simulink model "DVB_S2X_64APSK_Receiver_Sim"  (R2025b)
settings: Solver=VariableStepAuto  StartTime=0.0  StopTime=10.0  RelTol=1e-3
libraries: simulink x1
settings Model: Creator=vaggelis  LastModifiedBy=vaggelis

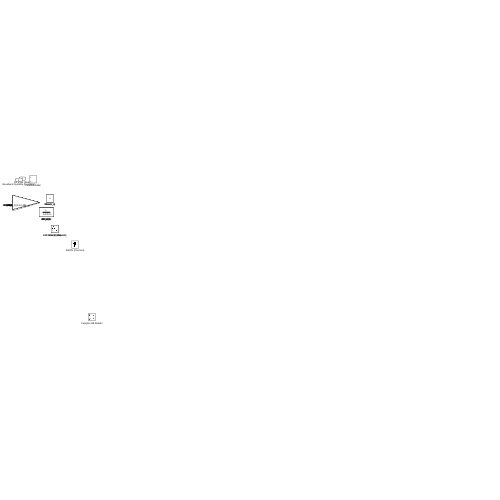
[thumbnail: Simulink's stored preview of the top-level diagram]
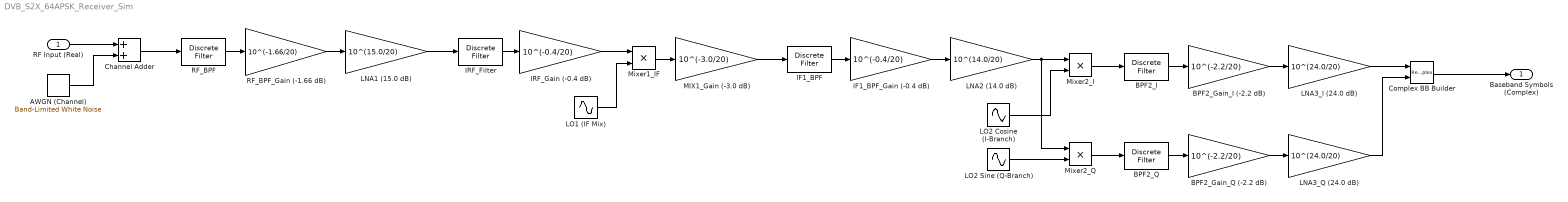
== system DVB_S2X_64APSK_Receiver_Sim ==
  RF Input (Real) : Inport
  AWGN (Channel) : simulink/Sources/Band-Limited White Noise  Cov=0.01  Ts=0.1  seed=[23341]
  BPF2_Gain_I (-2.2 dB) : Gain  Gain=10^(-2.2/20)
  BPF2_Gain_Q (-2.2 dB) : Gain  Gain=10^(-2.2/20)
  BPF2_I : DiscreteFilter
  BPF2_Q : DiscreteFilter
  Channel Adder : Sum
  Complex BB Builder : RealImagToComplex
  IF1_BPF : DiscreteFilter
  IF1_BPF_Gain (-0.4 dB) : Gain  Gain=10^(-0.4/20)
  IRF_Filter : DiscreteFilter
  IRF_Gain (-0.4 dB) : Gain  Gain=10^(-0.4/20)
  LNA1 (15.0 dB) : Gain  Gain=10^(15.0/20)
  LNA2 (14.0 dB) : Gain  Gain=10^(14.0/20)
  LNA3_I (24.0 dB) : Gain  Gain=10^(24.0/20)
  LNA3_Q (24.0 dB) : Gain  Gain=10^(24.0/20)
  LO1 (IF Mix) : Sin  Amplitude=2  Frequency=2*pi*22.5e9  SampleTime=0
  LO2 Cosine (I-Branch) : Sin  Amplitude=2  Frequency=2*pi*1.5e9  SampleTime=0
  LO2 Sine (Q-Branch) : Sin  Amplitude=-2  Frequency=2*pi*1.5e9  Phase=pi/2  SampleTime=0
  MIX1_Gain (-3.0 dB) : Gain  Gain=10^(-3.0/20)
  Mixer1_IF : Product
  Mixer2_I : Product
  Mixer2_Q : Product
  RF_BPF : DiscreteFilter
  RF_BPF_Gain (-1.66 dB) : Gain  Gain=10^(-1.66/20)
  Baseband Symbols (Complex) : Outport
  wires:
  Complex BB Builder/1 -> Baseband Symbols (Complex)/1
  BPF2_Gain_Q (-2.2 dB)/1 -> LNA3_Q (24.0 dB)/1
  BPF2_Gain_I (-2.2 dB)/1 -> LNA3_I (24.0 dB)/1
  BPF2_Q/1 -> BPF2_Gain_Q (-2.2 dB)/1
  Mixer2_I/1 -> BPF2_I/1
  Mixer2_Q/1 -> BPF2_Q/1
  LO2 Sine (Q-Branch)/1 -> Mixer2_Q/2
  LNA3_Q (24.0 dB)/1 -> Complex BB Builder/2
  LO2 Cosine (I-Branch)/1 -> Mixer2_I/2
  LNA2 (14.0 dB)/1 -> Mixer2_Q/1, Mixer2_I/1
  RF Input (Real)/1 -> Channel Adder/1
  AWGN (Channel)/1 -> Channel Adder/2
  MIX1_Gain (-3.0 dB)/1 -> IF1_BPF/1
  Channel Adder/1 -> RF_BPF/1
  RF_BPF/1 -> RF_BPF_Gain (-1.66 dB)/1
  RF_BPF_Gain (-1.66 dB)/1 -> LNA1 (15.0 dB)/1
  LO1 (IF Mix)/1 -> Mixer1_IF/2
  LNA1 (15.0 dB)/1 -> IRF_Filter/1
  IRF_Filter/1 -> IRF_Gain (-0.4 dB)/1
  Mixer1_IF/1 -> MIX1_Gain (-3.0 dB)/1
  IF1_BPF/1 -> IF1_BPF_Gain (-0.4 dB)/1
  LNA3_I (24.0 dB)/1 -> Complex BB Builder/1
  IRF_Gain (-0.4 dB)/1 -> Mixer1_IF/1
  BPF2_I/1 -> BPF2_Gain_I (-2.2 dB)/1
  IF1_BPF_Gain (-0.4 dB)/1 -> LNA2 (14.0 dB)/1
